simulink model "CO_APOD5levelCHBInverter"  (R2023a)
settings: Solver=VariableStepAuto  StartTime=0.0  StopTime=0.04  RelTol=1e-3
libraries: spsIGBTDiodeLib x8, simulink x6, spsDCVoltageSourceLib x2, spsSeriesRLCBranchLib x1, spsVoltageMeasurementLib x1, sps_lib x1
settings Model: Creator=User  LastModifiedBy=User

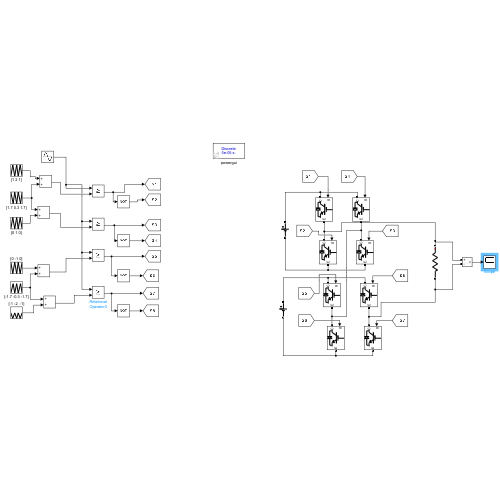
[thumbnail: Simulink's stored preview of the top-level diagram]
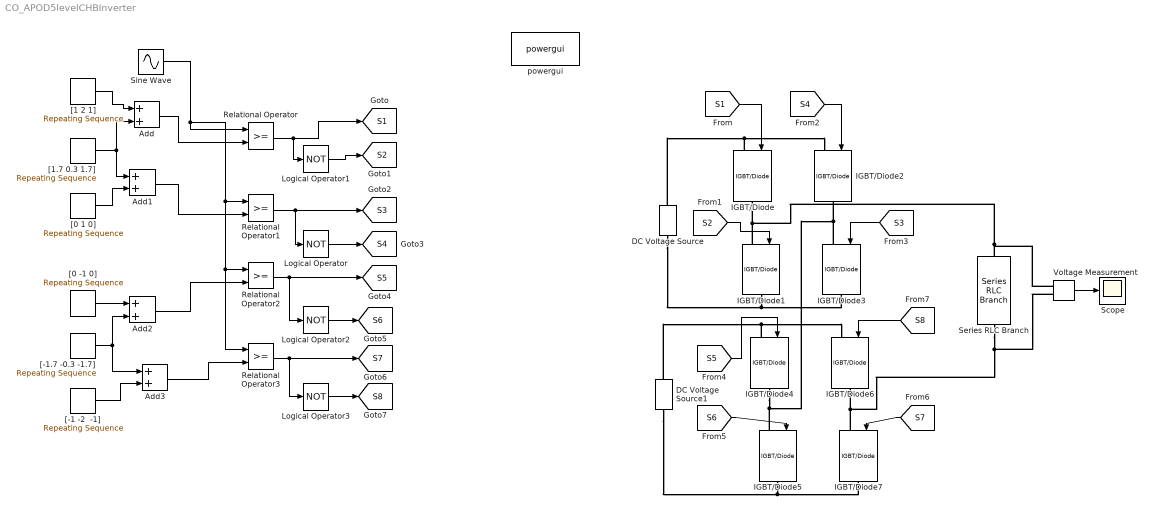
== system CO_APOD5levelCHBInverter ==
  Add{,1..3} (4 alike) : Sum
  DC Voltage Source : spsDCVoltageSourceLib/DC Voltage Source  Amplitude=100  Measurements=None
  DC Voltage Source1 : spsDCVoltageSourceLib/DC Voltage Source  Amplitude=100  Measurements=None
  IGBT/Diode{,1..7} (8 alike) : spsIGBTDiodeLib/IGBT//Diode  Ron=1e-3  Rs=1e5  Cs=inf  Measurements=off
  Logical Operator{,1..3} (4 alike) : Logic  Operator=NOT  AllPortsSameDT=off  OutDataTypeStr=boolean
  Relational Operator{,1..3} (4 alike) : RelationalOperator  OutDataTypeStr=boolean  RndMeth=Simplest  InputSameDT=off
  Scope : Scope
  Series RLC Branch : spsSeriesRLCBranchLib/Series RLC Branch  LConnTagsString=__new0  RConnTagsString=__new0  BranchType=R  Resistance=10  Inductance=1e-3  SetiL0=off  InitialCurrent=0  Capacitance=1e-6  Setx0=off  InitialVoltage=0  Measurements=None
  Sine Wave : Sin  Amplitude=2  Frequency=2*pi*50  SampleTime=0
  Voltage Measurement : spsVoltageMeasurementLib/Voltage Measurement  PhasorSimulation=off  OutputType=Complex  PSBequivalent=0
  "[-1 -2  -1]" : simulink/Sources/Repeating Sequence  rep_seq_t=[0 0.5 1]/1000  rep_seq_y="[-1 -2  -1]"
  "[-1.7 -0.3 -1.7]" : simulink/Sources/Repeating Sequence  rep_seq_t=[0.0010 0.6010 1.020]/1000  rep_seq_y=[-1.7 -0.3 -1.7]
  "[0 -1 0]" : simulink/Sources/Repeating Sequence  rep_seq_t=[0 0.5 1]/1000  rep_seq_y=[0 -1 0]
  "[0 1 0]" : simulink/Sources/Repeating Sequence  rep_seq_t=[0 0.5 1]/1000  rep_seq_y=[0 1 0]
  "[1 2 1]" : simulink/Sources/Repeating Sequence  rep_seq_t=[0 0.5 1]/1000  rep_seq_y=[1 2 1]
  "[1.7 0.3 1.7]" : simulink/Sources/Repeating Sequence  rep_seq_t=[0.0010 0.6010 1.020]/1000  rep_seq_y=[1.7 0.3 1.7]
  powergui : sps_lib/powergui  Priority=1  SimulationMode=Discrete  SampleTime=50e-6  frequency=60  Iterations=50  frequencyindice=0  Pbase=100e6  ErrMax=1e-4  UnitsV=kV  UnitsW=MW  buscounter=0  FunctionMessages=off  echomessages=off  EnableUseOfTLC=off  CurrentSourceSwitches=off  DisableSnubberDevices=off  DisableRonSwitches=off  DisableVfSwitches=off  DisplayEquations=off  AutomaticDiscreteSolvers=off  SolverType=Tustin/Backward Euler (TBE)  Interpol=off  ExternalGateDelay=off  methode=off  Ts=100  x0status=blocks  SPID=on  SwTol=0  HookPort=off  NonlinearTolerance=1e-4  nMaxIteration=100  ContinueOnMaxIteration=off  RestoreLinks=warning  ResistiveCurrentMeasurement=off  Frange=[0:2:500]  Ylog=off  Xlog=on  ShowGrid=off  save=off  variable=ZData  structure=0  ZoomFFT=off  StartTime=0.0  cycles=1  DisplayStyle=1  fundamental=60  FreqAxis=off  MaxFrequency=1000  frequencyindicesteady=1  RmsSteady=1  display=off
  tag scope: S1=global, S2=global, S3=global, S4=global, S5=global, S6=global, S7=global, S8=global
  wires:
  Relational Operator/1 -> Logical Operator1/1, [S1]
  [S6] -> IGBT/Diode5/1
  [S1] -> IGBT/Diode/1
  "[1.7 0.3 1.7]"/1 -> Add/2, Add1/1
  [S3] -> IGBT/Diode3/1
  [S7] -> IGBT/Diode7/1
  Relational Operator2/1 -> Logical Operator2/1, [S5]
  "[-1.7 -0.3 -1.7]"/1 -> Add2/2, Add3/1
  Voltage Measurement/1 -> Scope/1
  [S8] -> IGBT/Diode6/1
  Logical Operator2/1 -> [S6]
  Logical Operator1/1 -> [S2]
  [S2] -> IGBT/Diode1/1
  Logical Operator3/1 -> [S8]
  Relational Operator1/1 -> Logical Operator/1, [S3]
  Relational Operator3/1 -> Logical Operator3/1, [S7]
  [S4] -> IGBT/Diode2/1
  Logical Operator/1 -> [S4]
  [S5] -> IGBT/Diode4/1
  Add/1 -> Relational Operator/2
  "[0 1 0]"/1 -> Add1/2
  "[1 2 1]"/1 -> Add/1
  Sine Wave/1 -> Relational Operator3/1, Relational Operator2/1, Relational Operator1/1, Relational Operator/1
  Add1/1 -> Relational Operator1/2
  Add2/1 -> Relational Operator2/2
  "[0 -1 0]"/1 -> Add2/1
  "[-1 -2  -1]"/1 -> Add3/2
  Add3/1 -> Relational Operator3/2
  connections:
  IGBT/Diode5/LConn1 -- IGBT/Diode4/RConn1 -- IGBT/Diode2/RConn1 -- IGBT/Diode3/LConn1
  IGBT/Diode/LConn1 -- IGBT/Diode2/LConn1 -- DC Voltage Source/RConn1
  Series RLC Branch/RConn1 -- IGBT/Diode6/RConn1 -- IGBT/Diode7/LConn1 -- Voltage Measurement/LConn2
  IGBT/Diode1/RConn1 -- IGBT/Diode3/RConn1 -- DC Voltage Source/LConn1
  IGBT/Diode5/RConn1 -- IGBT/Diode7/RConn1 -- DC Voltage Source1/LConn1
  Series RLC Branch/LConn1 -- IGBT/Diode/RConn1 -- IGBT/Diode1/LConn1 -- Voltage Measurement/LConn1
  IGBT/Diode4/LConn1 -- IGBT/Diode6/LConn1 -- DC Voltage Source1/RConn1
